simulink model "BTC_sfun"  (R2024b)
settings: Solver=FixedStepDiscrete  StartTime=0.0  StopTime=inf  RelTol=1e-3  EnableMultiTasking=on
values from neighbouring files (symbols this model uses):
  btcc_ambient_temp_highth = 45    [BTC_init.m]
  btcc_ambient_temp_lowth = -30    [BTC_init.m]
  btcc_cell_temp_diffth = 5    [BTC_init.m]
  btcc_full_soc = 95    [BTC_init.m]
  btcc_Ki = 0.5    [BTC_init.m]
  btcc_Kp = 2    [BTC_init.m]
  btcc_max_temp_highth = 40    [BTC_init.m]
  btcc_max_temp_lowth = 35    [BTC_init.m]
  btcc_min_temp_highth = 25    [BTC_init.m]
  btcc_min_temp_lowth = 20    [BTC_init.m]
  btcc_number_in_series = 40    [BTC_init.m]
  btcc_pack_in_parallel = 1    [BTC_init.m]
  btck_stepSize = 0.1    [BTC_init.m]
settings Model: TunableVars=btcc_Ki,btcc_Kp,btcc_ambient_temp_highth,btcc_ambient_temp_lowth,btcc_cell_temp_diffth,btcc_full_soc,btcc_max_temp_highth,btcc_max_temp_lowth,btcc_min_temp_highth,btcc_min_temp_lowth,btcc_number_in_series,btcc_pack_in_parallel,btck_stepSize  TunableVarsStorageClass=Auto,Auto,Auto,Auto,Auto,Auto,Auto,Auto,Auto,Auto,Auto,Auto,Auto  TunableVarsTypeQualifier=,,,,,,,,,,,,  Creator=nctzv8  LastModifiedBy=voillat
settings ConfigSet: Description=OpenECU configuration set for code generation under RTW-EC.
settings SolverCC: AlgebraicLoopSolver=TrustRegion  PositivePriorityOrder=on
settings DataIOCC: LimitDataPoints=on  SaveFormat=Array  SignalLoggingSaveFormat=ModelDataLogs
settings OptimizationCC: DefaultParameterBehavior=Inlined  InlineInvariantSignals=on  ExpressionDepthLimit=2147483647  StateBitsets=on  DataBitsets=on  ZeroExternalMemoryAtStartup=off  ZeroInternalMemoryAtStartup=off  NoFixptDivByZeroProtection=on  EfficientFloat2IntCast=on  LifeSpan=1  EfficientTunableParamExpr=on
settings DebuggingCC: SaveWithParameterizedLinksMsg=none  SignalResolutionControl=TryResolveAllWithWarning  MultiTaskDSMMsg=warning  MultiTaskCondExecSysMsg=none  SingleTaskRateTransMsg=error  CheckMatrixSingularityMsg=warning  VectorMatrixConversionMsg=warning  SignalLabelMismatchMsg=warning  UnconnectedInputMsg=warning  UnconnectedOutputMsg=warning  UnconnectedLineMsg=warning  AllowSymbolicDim=off  StateNameClashWarn=warning  SFUnexpectedBacktrackingDiag=warning  SFNoUnconditionalDefaultTransitionDiag=warning  SFExecutionAtInitializationDiag=none  ArithmeticOperatorsInVariantConditions=warning
settings HardwareCC: ProdBitPerPointer=32  ProdBitPerSizeT=32  ProdBitPerPtrDiffT=32  ProdLargestAtomicInteger=Long  ProdLargestAtomicFloat=Double  ProdEndianess=BigEndian  ProdWordSize=32  ProdHWDeviceType=Freescale->32-bit PowerPC  TargetIntDivRoundTo=Zero  TargetEndianess=BigEndian  TargetHWDeviceType=Freescale->32-bit PowerPC  ProdEqTarget=off
settings ModelReferenceCC: EnableRefExpFcnMdlSchedulingChecks=on  PropagateSignalLabelsOutOfModel=off
settings SFSimCC: SimUseLocalCustomCode=off  MATLABDynamicMemAlloc=off  CustomCodeUndefinedFunction=UseInterfaceOnly
settings RTWCC: Description=OpenECU Platform Target (ERT, optimised floating-point code)  SystemTargetFile=openecu_ert.tlc  MakeCommand=make_rtw optimized_floating_point=1  TemplateMakefile=openecu_ert_r2015b_64.tmf  RetainRTWFile=on  RTWUseLocalCustomCode=off  IncludeHyperlinkInReport=on  GPUComputeCapability=3.5
settings CodeAppCC: ForceParamTrailComments=on  IgnoreCustomStorageClasses=off  SimulinkDataObjDesc=on  CustomSymbolStrType=$N$R$M  InsertBlockDesc=on  StateflowObjectComments=on  InternalIdentifier=Classic
settings STFCustomTargetCC: TargetLibSuffix=.a  GenerateSampleERTMain=on  IncludeMdlTerminateFcn=off  CombineOutputUpdateFcns=on  IncludeFileDelimiter=UseQuote  ERTCustomFileBanners=on  SupportContinuousTime=off  RemoveResetFunc=on  MATLABClassNameForMDSCustomization=Simulink.SoftwareTarget.ERTCustomization  SystemTargetFile=openecu_ert.tlc
settings ERTTargetCC: MultiwordLength=2048  GenerateSampleERTMain=on  ParMdlRefBuildCompliant=off  CompOptLevelCompliant=off  ConcurrentExecutionCompliant=off  IncludeMdlTerminateFcn=off  IncludeFileDelimiter=UseQuote  SupportNonInlinedSFcns=on  ModelStepFunctionPrototypeControlCompliant=off  CPPClassGenCompliant=off  UseToolchainInfoCompliant=off  ExtModeMexFile=noextcomm  ERTSrcFileBannerTemplate=oe_code_c_template.cgt  ERTHdrFileBannerTemplate=oe_code_h_template.cgt  ERTDataSrcFileTemplate=oe_data_c_template.cgt  ERTDataHdrFileTemplate=oe_data_h_template.cgt  ERTCustomFileTemplate=example_file_process.tlc  GlobalDataDefinition=InSeparateSourceFile  GlobalDataReference=InSeparateHeaderFile  ConvertIfToSwitch=off  SuppressUnreachableDefaultCases=off  EnableUserReplacementTypes=on  DynamicArrayContainerType=coder::array
settings ConfigComp: CovMetricSettings=dw  CovSaveCumulativeToWorkspaceVar=on  CovSaveSingleToWorkspaceVar=on  CovExternalEMLEnable=off

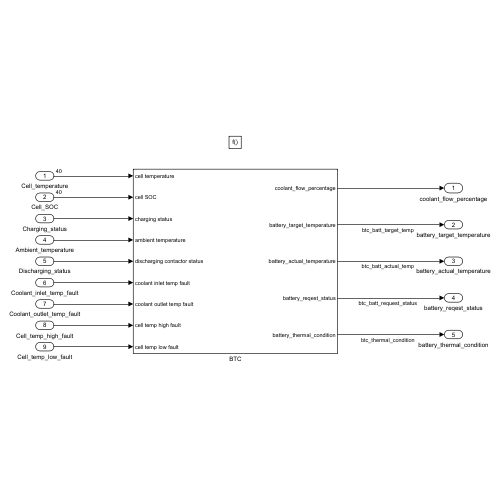
[thumbnail: Simulink's stored preview of the top-level diagram]
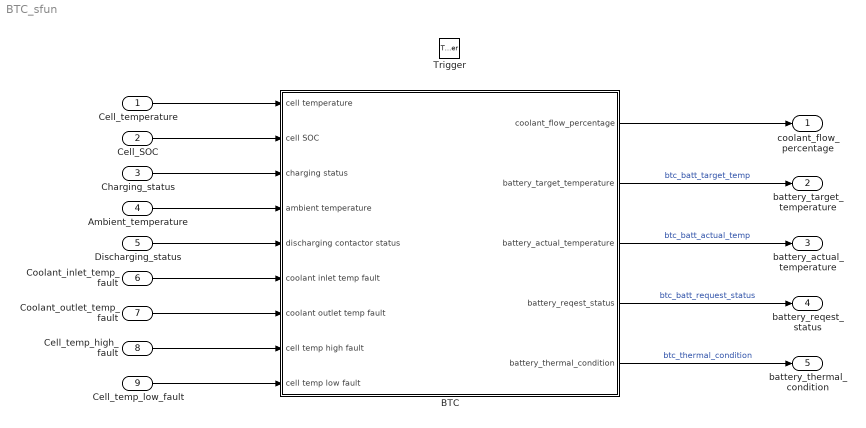
== system BTC_sfun ==
  Cell_temperature : Inport  PortDimensions=40
  Cell_SOC : Inport  Port=2  PortDimensions=40
  Charging_status : Inport  Port=3
  Ambient_temperature : Inport  Port=4
  Discharging_status : Inport  Port=5
  Coolant_inlet_temp_fault : Inport  Port=6
  Coolant_outlet_temp_fault : Inport  Port=7
  Cell_temp_high_fault : Inport  Port=8
  Cell_temp_low_fault : Inport  Port=9
  Trigger : TriggerPort  TriggerType=function-call  VariantControl=(inherit)  PortDimensions=1
  BTC : Subsystem  mask{prm_to_disp=[1..10], sfcnParam1=btcc_Ki, sfcnParam2=btcc_Kp, sfcnParam3=btcc_ambient_temp_highth, sfcnParam4=btcc_ambient_temp_lowth, sfcnParam5=btcc_cell_temp_diffth, sfcnParam6=btcc_full_soc, sfcnParam7=btcc_max_temp_highth, sfcnParam8=btcc_max_temp_lowth, sfcnParam9=btcc_min_temp_highth, sfcnParam10=btcc_min_temp_lowth, sfcnParam11=btcc_number_in_series, sfcnParam12=btcc_pack_in_parallel, sfcnParam13=btck_stepSize}
      mask prompts: prm_to_disp "Display S-function Parameters:"; sfcnParam1 "btcc_Ki:"; sfcnParam2 "btcc_Kp:"; sfcnParam3 "btcc_ambient_temp_highth:"; sfcnParam4 "btcc_ambient_temp_lowth:"; sfcnParam5 "btcc_cell_temp_diffth:"; sfcnParam6 "btcc_full_soc:"; sfcnParam7 "btcc_max_temp_highth:"; sfcnParam8 "btcc_max_temp_lowth:"; sfcnParam9 "btcc_min_temp_highth:"; sfcnParam10 "btcc_min_temp_lowth:"; sfcnParam11 "btcc_number_in_series:"; sfcnParam12 "btcc_pack_in_parallel:"; sfcnParam13 "btck_stepSize:"
      mask help: Simulink:masks:GenSFuncDesc_MD
      mask Help: eval('feval(''rtwprivate'',''rtwhelpview'',''rtw_sfcn_block'')');
      mask TypeOptions prm_to_disp: [1..10] | [11..13]
      mask Callback prm_to_disp: slmaskprmdispcntrl(gcbh)
  coolant_flow_percentage : Outport
  battery_target_temperature : Outport  Port=2
  battery_actual_temperature : Outport  Port=3
  battery_reqest_status : Outport  Port=4
  battery_thermal_condition : Outport  Port=5
  wires:
  Cell_temperature/1 -> BTC/1(cell temperature)
  Cell_SOC/1 -> BTC/2(cell SOC)
  Charging_status/1 -> BTC/3(charging status)
  Ambient_temperature/1 -> BTC/4(ambient temperature)
  Discharging_status/1 -> BTC/5(discharging contactor status)
  Coolant_inlet_temp_fault/1 -> BTC/6(coolant inlet temp fault)
  Coolant_outlet_temp_fault/1 -> BTC/7(coolant outlet temp fault)
  Cell_temp_high_fault/1 -> BTC/8(cell temp high fault)
  Cell_temp_low_fault/1 -> BTC/9(cell temp low fault)
  BTC/1(coolant_flow_percentage) -> coolant_flow_percentage/1
  BTC/2(battery_target_temperature) -> battery_target_temperature/1  "btc_batt_target_temp"
  BTC/3(battery_actual_temperature) -> battery_actual_temperature/1  "btc_batt_actual_temp"
  BTC/4(battery_reqest_status) -> battery_reqest_status/1  "btc_batt_request_status"
  BTC/5(battery_thermal_condition) -> battery_thermal_condition/1  "btc_thermal_condition"

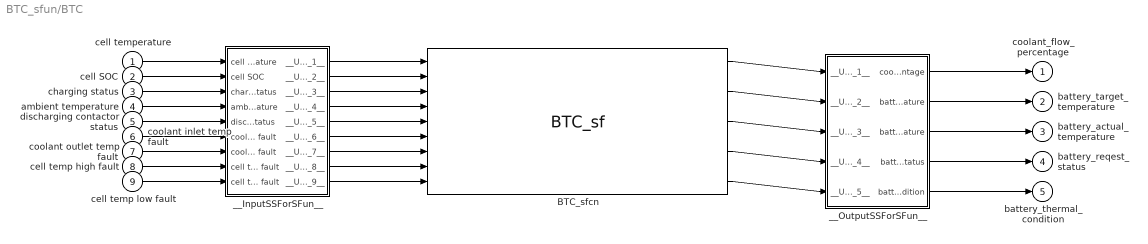
== system BTC_sfun/BTC ==
  cell temperature : Inport
  cell SOC : Inport  Port=2
  charging status : Inport  Port=3
  ambient temperature : Inport  Port=4
  discharging contactor status : Inport  Port=5
  coolant inlet temp fault : Inport  Port=6
  coolant outlet temp fault : Inport  Port=7
  cell temp high fault : Inport  Port=8  OutDataTypeStr=uint8
  cell temp low fault : Inport  Port=9  OutDataTypeStr=uint8
  BTC_sfcn : S-Function  FunctionName=BTC_sf  Parameters=sfcnParam1, sfcnParam2, sfcnParam3, sfcnParam4, sfcnParam5, sfcnParam6, sfcnParam7, sfcnParam8, sfcnParam9, sfcnParam10, sfcnParam11, sfcnParam12, sfcnParam13  SFunctionModules=""  SFunctionDeploymentMode=off  EnableBusSupport=off  mask{rtw_sf_name=BTC_sf, showVar=off, prm_to_disp=[1..10], sfcnParam1=sfcnParam1, sfcnParam2=sfcnParam2, sfcnParam3=sfcnParam3, sfcnParam4=sfcnParam4, sfcnParam5=sfcnParam5, sfcnParam6=sfcnParam6, sfcnParam7=sfcnParam7, sfcnParam8=sfcnParam8, sfcnParam9=sfcnParam9, sfcnParam10=sfcnParam10, sfcnParam11=sfcnParam11, sfcnParam12=sfcnParam12, sfcnParam13=sfcnParam13}
      mask prompts: rtw_sf_name "Simulink:masks:GenSFuncName_MP"; showVar "Simulink:masks:GenSFuncShowModuleList_MP"; prm_to_disp "Display S-function Parameters:"; sfcnParam1 "btcc_Ki:"; sfcnParam2 "btcc_Kp:"; sfcnParam3 "btcc_ambient_temp_highth:"; sfcnParam4 "btcc_ambient_temp_lowth:"; sfcnParam5 "btcc_cell_temp_diffth:"; sfcnParam6 "btcc_full_soc:"; sfcnParam7 "btcc_max_temp_highth:"; sfcnParam8 "btcc_max_temp_lowth:"; sfcnParam9 "btcc_min_temp_highth:"; sfcnParam10 "btcc_min_temp_lowth:"; sfcnParam11 "btcc_number_in_series:"; sfcnParam12 "btcc_pack_in_parallel:"; sfcnParam13 "btck_stepSize:"
      mask help: Simulink:masks:GenSFuncDesc_MD
      mask init:
      | displist = '';
      | if ~strcmp(get_param(gcb, 'FunctionName'), rtw_sf_name);
      |   set_param(gcb, 'FunctionName', rtw_sf_name);
      | end
      | % Check if we are generating code
      | rtw_mode = false;
      | if strcmpi(get_param(bdroot(gcb),'SimulationStatus'),'Initializing')
      | 	rtw_mode = strcmpi(get_param(bdroot(gcb),'BuildingRTWCode'),'on') && ...
      | 		~strcmpi(get_param(bdroot(gcb),'TargetStyle'),'SimulationTarget');
      | end
      | if showVar || rtw_mode
      | 	if exist('rtwsfunc') == 2 | exist('rtwsfunc') == 6
      | 		tmplist = rtwsfunc(rtw_sf_name,gcb);
      | 		tmplist = DAStudio.message('Simulink:masks:GenSFuncListOfModules_IC', tmplist);
      | 	elseif showVar
      | 		tmplist1 = DAStudio.message('Simulink:masks:GenSFuncListOfModules_IC', '');
      |         tmplist2 = DAStudio.message('Simulink:masks:GenSFuncNotLicensed_IC');
      |         tmplist = [tmplist1 tmplist2];
      |  	end
      | end
      | if showVar
      |   displist = tmplist;
      | end
      settings: CopyFcn=|
      | if ~strcmp(get_param(gcb,'Linkstatus'),'none') && ...
      | ~strcmp(get_param(gcb,'Linkstatus'),'implicit')
      |   set_param(gcb,'LinkStatus','none');
      | end
      mask Help: eval('feval(''rtwprivate'',''rtwhelpview'',''rtw_sfcn_block'')');
      mask TypeOptions prm_to_disp: [1..10] | [11..13]
      mask Callback prm_to_disp: slmaskprmdispcntrl(gcbh)
      mask Display:
      | port_label('input',1,'cell temperature');
      | port_label('input',2,'cell SOC');
      | port_label('input',3,'charging status');
      | port_label('input',4,'ambient temperature');
      | port_label('input',5,'discharging contactor status');
      | port_label('input',6,'coolant inlet temp fault');
      | port_label('input',7,'coolant outlet temp fault');
      | port_label('input',8,'cell temp high fault');
      | port_label('input',9,'cell temp low fault');
      | port_label('output',1,'coolant_flow_percentage');
      | port_label('output',2,'battery_target_temperature');
      | port_label('output',3,'battery_actual_temperature');
      | port_label('output',4,'battery_reqest_status');
      | port_label('output',5,'battery_thermal_condition');
  __InputSSForSFun__ : Subsystem
  __OutputSSForSFun__ : Subsystem
  coolant_flow_percentage : Outport
  battery_target_temperature : Outport  Port=2
  battery_actual_temperature : Outport  Port=3
  battery_reqest_status : Outport  Port=4
  battery_thermal_condition : Outport  Port=5
  wires:
  cell temperature/1 -> __InputSSForSFun__/1(cell temperature)
  cell SOC/1 -> __InputSSForSFun__/2(cell SOC)
  charging status/1 -> __InputSSForSFun__/3(charging status)
  ambient temperature/1 -> __InputSSForSFun__/4(ambient temperature)
  discharging contactor status/1 -> __InputSSForSFun__/5(discharging contactor status)
  coolant inlet temp fault/1 -> __InputSSForSFun__/6(coolant inlet temp fault)
  coolant outlet temp fault/1 -> __InputSSForSFun__/7(coolant outlet temp fault)
  cell temp high fault/1 -> __InputSSForSFun__/8(cell temp high fault)
  cell temp low fault/1 -> __InputSSForSFun__/9(cell temp low fault)
  __InputSSForSFun__/1(__UniqueOutportName__1__) -> BTC_sfcn/1
  __InputSSForSFun__/2(__UniqueOutportName__2__) -> BTC_sfcn/2
  __InputSSForSFun__/3(__UniqueOutportName__3__) -> BTC_sfcn/3
  __InputSSForSFun__/4(__UniqueOutportName__4__) -> BTC_sfcn/4
  __InputSSForSFun__/5(__UniqueOutportName__5__) -> BTC_sfcn/5
  __InputSSForSFun__/6(__UniqueOutportName__6__) -> BTC_sfcn/6
  __InputSSForSFun__/7(__UniqueOutportName__7__) -> BTC_sfcn/7
  __InputSSForSFun__/8(__UniqueOutportName__8__) -> BTC_sfcn/8
  __InputSSForSFun__/9(__UniqueOutportName__9__) -> BTC_sfcn/9
  BTC_sfcn/1 -> __OutputSSForSFun__/1(__UniqueInportName__1__)
  BTC_sfcn/2 -> __OutputSSForSFun__/2(__UniqueInportName__2__)
  BTC_sfcn/3 -> __OutputSSForSFun__/3(__UniqueInportName__3__)
  BTC_sfcn/4 -> __OutputSSForSFun__/4(__UniqueInportName__4__)
  BTC_sfcn/5 -> __OutputSSForSFun__/5(__UniqueInportName__5__)
  __OutputSSForSFun__/1(coolant_flow_percentage) -> coolant_flow_percentage/1
  __OutputSSForSFun__/2(battery_target_temperature) -> battery_target_temperature/1
  __OutputSSForSFun__/3(battery_actual_temperature) -> battery_actual_temperature/1
  __OutputSSForSFun__/4(battery_reqest_status) -> battery_reqest_status/1
  __OutputSSForSFun__/5(battery_thermal_condition) -> battery_thermal_condition/1

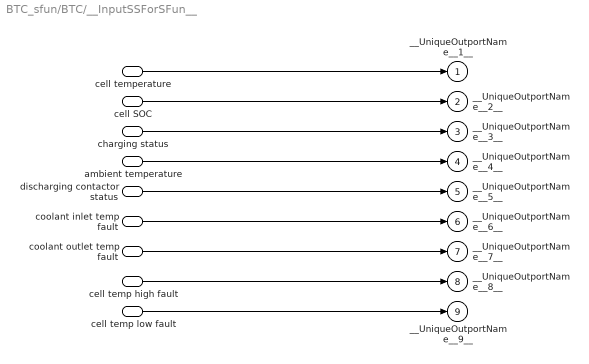
== system BTC_sfun/BTC/__InputSSForSFun__ ==
  cell temperature : Inport
  cell SOC : Inport  Port=2
  charging status : Inport  Port=3
  ambient temperature : Inport  Port=4
  discharging contactor status : Inport  Port=5
  coolant inlet temp fault : Inport  Port=6
  coolant outlet temp fault : Inport  Port=7
  cell temp high fault : Inport  Port=8  OutDataTypeStr=uint8
  cell temp low fault : Inport  Port=9  OutDataTypeStr=uint8
  __UniqueOutportName__1__ : Outport
  __UniqueOutportName__2__ : Outport  Port=2
  __UniqueOutportName__3__ : Outport  Port=3
  __UniqueOutportName__4__ : Outport  Port=4
  __UniqueOutportName__5__ : Outport  Port=5
  __UniqueOutportName__6__ : Outport  Port=6
  __UniqueOutportName__7__ : Outport  Port=7
  __UniqueOutportName__8__ : Outport  Port=8
  __UniqueOutportName__9__ : Outport  Port=9
  wires:
  cell temperature/1 -> __UniqueOutportName__1__/1
  cell SOC/1 -> __UniqueOutportName__2__/1
  charging status/1 -> __UniqueOutportName__3__/1
  ambient temperature/1 -> __UniqueOutportName__4__/1
  discharging contactor status/1 -> __UniqueOutportName__5__/1
  coolant inlet temp fault/1 -> __UniqueOutportName__6__/1
  coolant outlet temp fault/1 -> __UniqueOutportName__7__/1
  cell temp high fault/1 -> __UniqueOutportName__8__/1
  cell temp low fault/1 -> __UniqueOutportName__9__/1

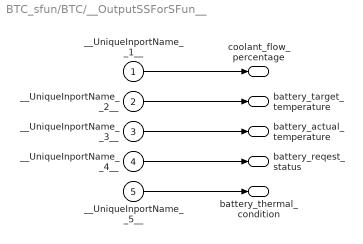
== system BTC_sfun/BTC/__OutputSSForSFun__ ==
  __UniqueInportName__1__ : Inport
  __UniqueInportName__2__ : Inport  Port=2
  __UniqueInportName__3__ : Inport  Port=3
  __UniqueInportName__4__ : Inport  Port=4
  __UniqueInportName__5__ : Inport  Port=5
  coolant_flow_percentage : Outport
  battery_target_temperature : Outport  Port=2
  battery_actual_temperature : Outport  Port=3
  battery_reqest_status : Outport  Port=4
  battery_thermal_condition : Outport  Port=5
  wires:
  __UniqueInportName__1__/1 -> coolant_flow_percentage/1
  __UniqueInportName__2__/1 -> battery_target_temperature/1
  __UniqueInportName__3__/1 -> battery_actual_temperature/1
  __UniqueInportName__4__/1 -> battery_reqest_status/1
  __UniqueInportName__5__/1 -> battery_thermal_condition/1
